simulink model "close_loop_system_obs"  (Simulink 7.7)
settings: Solver=ode45  StartTime=0.0  StopTime=10.0  RelTol=1e-3
values from neighbouring files (symbols this model uses):
  G = place((sys.a)', (sys.c(1,:))', Po)    [BE7_trame.m]
  Jt = 0.002    [BE7_trame.m]
  Kci = 1    [BE7_trame.m]
  Kcp = 1    [BE7_trame.m]
  Kcv = 0.0314    [BE7_trame.m]
  Ke = 0.2    [BE7_trame.m]
  Kg = 0.2    [BE7_trame.m]
  Le = 0.002    [BE7_trame.m]
  N = 300    [BE7_trame.m]
  Re = 2    [BE7_trame.m]
  sys = linmod('open_loop_system')    [BE7_trame.m]
libraries: simulink x2
settings Model: Creator=Anthony  LastModifiedBy=Anthony

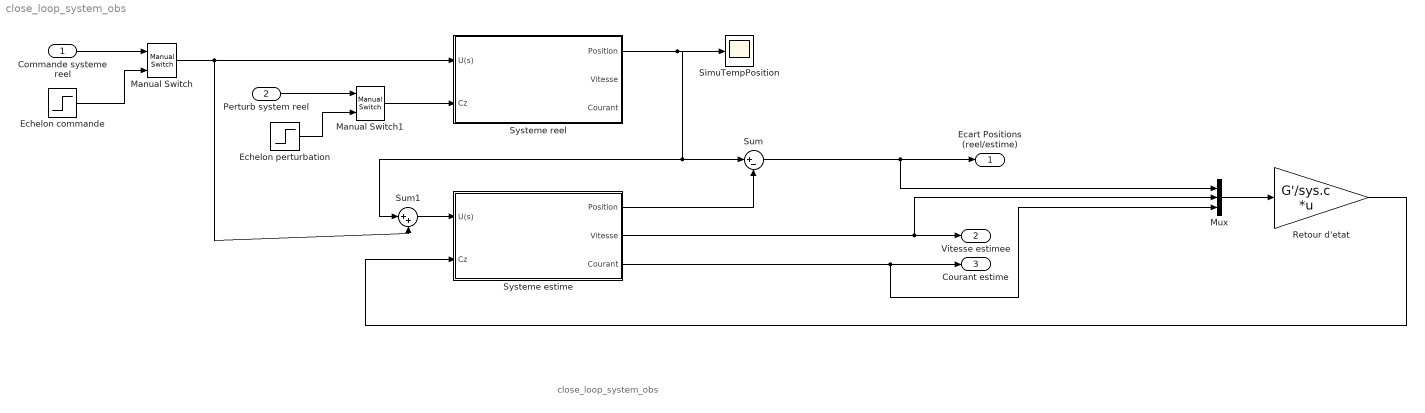
== system close_loop_system_obs ==
  note: close_loop_system_obs
  Commande systeme reel : Inport
  Perturb system reel : Inport  Port=2
  Echelon commande : Step  Time=0  After=100  SampleTime=0
  Echelon perturbation : Step  Time=5  After=5  SampleTime=0
  Manual Switch : simulink/Signal Routing/Manual Switch  SystemSampleTime=-1  sw=0  action=0  varsize=off
  Manual Switch1 : simulink/Signal Routing/Manual Switch  SystemSampleTime=-1  sw=0  action=0  varsize=off
  Mux : Mux  Inputs=3
  Retour d'etat : Gain  Gain=G'/sys.c  Multiplication=Matrix(K*u)
  SimuTempPosition : Scope
  Sum : Sum  Inputs=|+-
  Sum1 : Sum  Inputs=|++
  Systeme estime : Subsystem
  Systeme reel : Subsystem
  Ecart Positions (reel/estime) : Outport
  Vitesse estimee : Outport  Port=2
  Courant estime : Outport  Port=3
  wires:
  Systeme reel/1(Position) -> SimuTempPosition/1, Sum/1, Sum1/1
  Systeme estime/1(Position) -> Sum/2
  Systeme estime/3(Courant) -> Courant estime/1, Mux/3
  Sum/1 -> Ecart Positions (reel/estime)/1, Mux/1
  Systeme estime/2(Vitesse) -> Vitesse estimee/1, Mux/2
  Mux/1 -> Retour d'etat/1
  Retour d'etat/1 -> Systeme estime/2(Cz)
  Commande systeme reel/1 -> Manual Switch/1
  Manual Switch/1 -> Systeme reel/1(U(s)), Sum1/2
  Perturb system reel/1 -> Manual Switch1/1
  Manual Switch1/1 -> Systeme reel/2(Cz)
  Echelon perturbation/1 -> Manual Switch1/2
  Echelon commande/1 -> Manual Switch/2
  Sum1/1 -> Systeme estime/1(U(s))

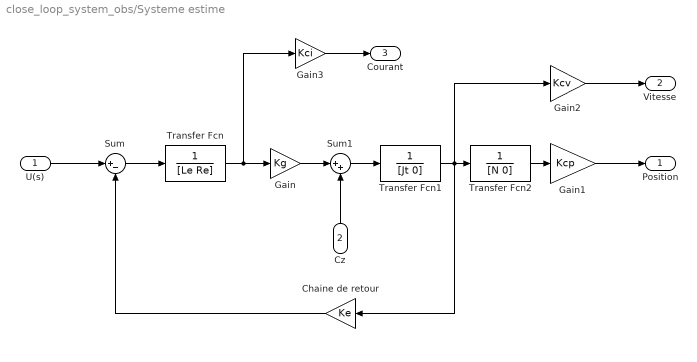
== system close_loop_system_obs/Systeme estime ==
  U(s) : Inport
  Cz : Inport  Port=2
  Chaine de retour : Gain  Gain=Ke
  Gain : Gain  Gain=Kg
  Gain1 : Gain  Gain=Kcp
  Gain2 : Gain  Gain=Kcv
  Gain3 : Gain  Gain=Kci
  Sum : Sum  Inputs=|+-
  Sum1 : Sum  Inputs=|++
  Transfer Fcn : TransferFcn  Denominator=[Le Re]
  Transfer Fcn1 : TransferFcn  Denominator=[Jt 0]
  Transfer Fcn2 : TransferFcn  Denominator=[N 0]
  Position : Outport
  Vitesse : Outport  Port=2
  Courant : Outport  Port=3
  wires:
  Gain1/1 -> Position/1
  Gain3/1 -> Courant/1
  Gain2/1 -> Vitesse/1
  Cz/1 -> Sum1/2
  U(s)/1 -> Sum/1
  Transfer Fcn2/1 -> Gain1/1
  Transfer Fcn1/1 -> Chaine de retour/1, Transfer Fcn2/1, Gain2/1
  Transfer Fcn/1 -> Gain/1, Gain3/1
  Sum/1 -> Transfer Fcn/1
  Sum1/1 -> Transfer Fcn1/1
  Gain/1 -> Sum1/1
  Chaine de retour/1 -> Sum/2

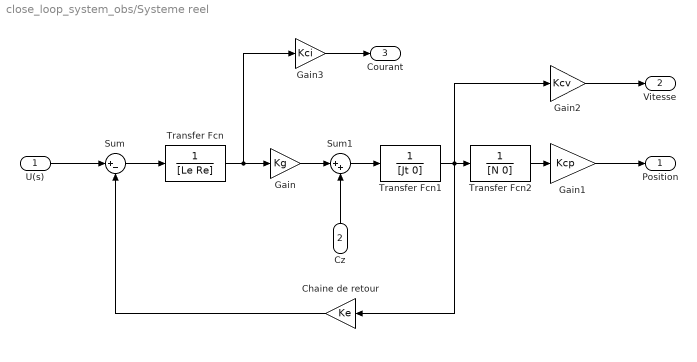
== system close_loop_system_obs/Systeme reel ==
  U(s) : Inport
  Cz : Inport  Port=2
  Chaine de retour : Gain  Gain=Ke
  Gain : Gain  Gain=Kg
  Gain1 : Gain  Gain=Kcp
  Gain2 : Gain  Gain=Kcv
  Gain3 : Gain  Gain=Kci
  Sum : Sum  Inputs=|+-
  Sum1 : Sum  Inputs=|++
  Transfer Fcn : TransferFcn  Denominator=[Le Re]
  Transfer Fcn1 : TransferFcn  Denominator=[Jt 0]
  Transfer Fcn2 : TransferFcn  Denominator=[N 0]
  Position : Outport
  Vitesse : Outport  Port=2
  Courant : Outport  Port=3
  wires:
  Gain1/1 -> Position/1
  Gain3/1 -> Courant/1
  Gain2/1 -> Vitesse/1
  Cz/1 -> Sum1/2
  U(s)/1 -> Sum/1
  Transfer Fcn2/1 -> Gain1/1
  Transfer Fcn1/1 -> Chaine de retour/1, Transfer Fcn2/1, Gain2/1
  Transfer Fcn/1 -> Gain/1, Gain3/1
  Sum/1 -> Transfer Fcn/1
  Sum1/1 -> Transfer Fcn1/1
  Gain/1 -> Sum1/1
  Chaine de retour/1 -> Sum/2
